simulink model "linear_interpolation_sim"  (R2020b)
settings: Solver=FixedStepAuto  StartTime=0.0  StopTime=stop_time  RelTol=1e-3
InitFcn:
  | linear_interpolation_sim_init
StopFcn:
  | linear_interpolation_sim_stop
values from neighbouring files (symbols this model uses):
  fs = 48e3    (= 48000)    [linear_interpolation_sim_init.m]
settings Model: Creator=t96f346  LastModifiedBy=conno
settings DataIOCC: ReturnWorkspaceOutputs=off

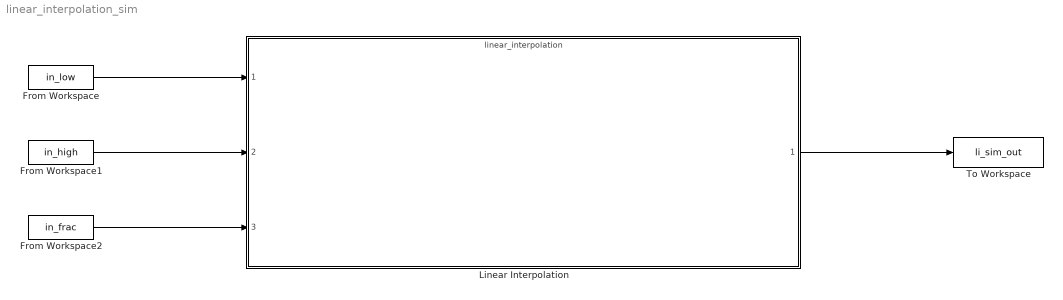
== system linear_interpolation_sim ==
  From Workspace : FromWorkspace  VariableName=in_low  SampleTime=1/fs
  From Workspace1 : FromWorkspace  VariableName=in_high  SampleTime=1/fs
  From Workspace2 : FromWorkspace  VariableName=in_frac  SampleTime=1/fs
  Linear Interpolation : ModelReference  ModelNameDialog=linear_interpolation.slx  SimulationMode=Normal  ModelReferenceVersion=1.3
  To Workspace : ToWorkspace  VariableName=li_sim_out  SampleTime=-1
  wires:
  From Workspace/1 -> Linear Interpolation/1
  From Workspace1/1 -> Linear Interpolation/2
  From Workspace2/1 -> Linear Interpolation/3
  Linear Interpolation/1 -> To Workspace/1
